simulink model "Test_Comparator"  (Simulink 8.1)
settings: Solver=ode45  StartTime=0.0  StopTime=10.0  RelTol=1e-3
libraries: Computer_Library x2
settings Model: Creator=uzivatel  LastModifiedBy=uzivatel
settings DataIOCC: SignalLoggingSaveFormat=Dataset
settings OptimizationCC: ExpressionDepthLimit=128
settings DebuggingCC: SolverPrmCheckMsg=none  FcnCallInpInsideContextMsg=EnableAllAsError
settings GRTTargetCC: CombineOutputUpdateFcns=on  GRTInterface=off

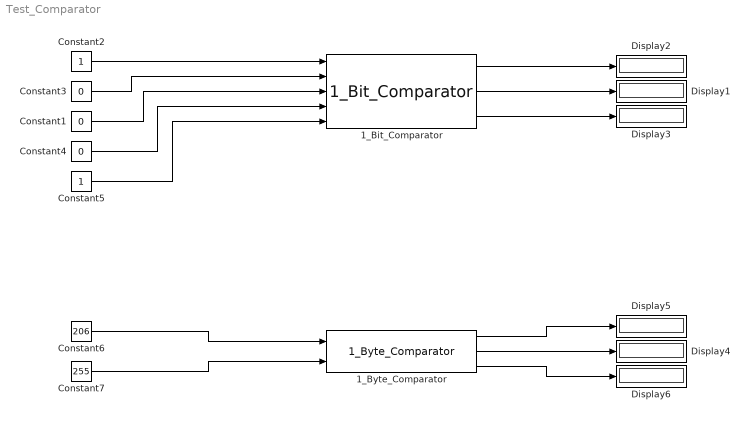
== system Test_Comparator ==
  1_Bit_Comparator : Computer_Library/Comparators/1_Bit_Comparator
  1_Byte_Comparator : Computer_Library/Comparators/1_Byte_Comparator
  Constant1 : Constant  Value=0  OutDataTypeStr=int16
  Constant2 : Constant  OutDataTypeStr=int16
  Constant3 : Constant  Value=0  OutDataTypeStr=int16
  Constant4 : Constant  Value=0  OutDataTypeStr=int16
  Constant5 : Constant  OutDataTypeStr=int16
  Constant6 : Constant  Value=206  OutDataTypeStr=int16
  Constant7 : Constant  Value=255  OutDataTypeStr=int16
  Display{1..6} (6 alike) : Display
  wires:
  Constant2/1 -> 1_Bit_Comparator/1
  Constant3/1 -> 1_Bit_Comparator/2
  Constant1/1 -> 1_Bit_Comparator/3
  Constant4/1 -> 1_Bit_Comparator/4
  Constant5/1 -> 1_Bit_Comparator/5
  1_Bit_Comparator/1 -> Display2/1
  1_Bit_Comparator/2 -> Display1/1
  1_Bit_Comparator/3 -> Display3/1
  1_Byte_Comparator/2 -> Display4/1
  1_Byte_Comparator/1 -> Display5/1
  1_Byte_Comparator/3 -> Display6/1
  Constant6/1 -> 1_Byte_Comparator/1
  Constant7/1 -> 1_Byte_Comparator/2
